simulink model "vipstabilize_fixpt_rowmajor"  (R2015b)
settings: Solver=FixedStepDiscrete  StartTime=0.0  StopTime=inf  RelTol=1e-3
undefined symbols (not defined in the file or in its folder): gray
libraries: visiontextngfix x3, visiongeotforms x2, visionsinks x2, vipmisc x1, dspvision x1, visionanalysis x1
Description:
  | Image stabilization demo.
settings Model: Tag="0  0  0  0  0  1"  FPTRunName=Active  ExtModeAutoUpdateStatusClock=off  Creator=The MathWorks, Inc.  LastModifiedBy=The MathWorks, Inc.
settings DataIOCC: SaveFormat=Array  SaveOutput=off  SaveTime=off  SignalLoggingName=logsOut
settings OptimizationCC: ExpressionDepthLimit=2147483647  InitFltsAndDblsToZero=on  BufferReusableBoundary=off
settings DebuggingCC: UnderspecifiedInitializationDetection=Classic  MergeDetectMultiDrivingBlocksExec=none  CheckExecutionContextPreStartOutputMsg=on  CheckExecutionContextRuntimeOutputMsg=on  SignalResolutionControl=TryResolveAllWithWarning  InheritedTsInSrcMsg=none  MultiTaskDSMMsg=warning  SigSpecEnsureSampleTimeMsg=none  ParameterPrecisionLossMsg=none  UnderSpecifiedDataTypeMsg=error  FcnCallInpInsideContextMsg=UseLocalSettings  BusObjectLabelMismatch=none  StateNameClashWarn=warning  StrictBusMsg=None
settings HardwareCC: ProdBitPerLong=40  ProdBitPerPointer=32  ProdLargestAtomicInteger=Integer  ProdLargestAtomicFloat=None  ProdWordSize=32  ProdHWDeviceType=TI C6000  TargetBitPerLong=64  TargetBitPerPointer=64  TargetLongLongMode=on  TargetIntDivRoundTo=Zero  TargetEndianess=LittleEndian  TargetWordSize=64  TargetHWDeviceType=MATLAB Host  ProdEqTarget=off
settings ModelReferenceCC: UpdateModelReferenceTargets=IfOutOfDate
settings GRTTargetCC: TargetFcnLib=ansi_tfl_tmw_new.mat  GeneratePreprocessorConditionals=Disable all  CombineOutputUpdateFcns=off  GRTInterface=on
settings ConfigComp: CovModelRefEnable=Off

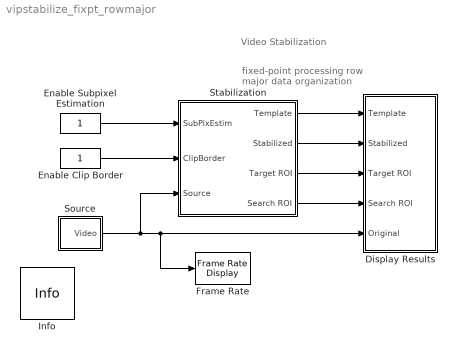
== system vipstabilize_fixpt_rowmajor ==
  note: Video Stabilization
  note: fixed-point processing
      | row major data organization
  Display Results : Subsystem
  Enable Clip Border : Constant  VectorParams1D=off  OutDataTypeStr=boolean
  Enable Subpixel Estimation : Constant  VectorParams1D=off  OutDataTypeStr=boolean
  Frame Rate : visionsinks/Frame Rate Display  UpdateRate=10
  Info : vipmisc/Info  SystemSampleTime=-1
  Source : Subsystem
  Stabilization : Subsystem  mask(Stabilization){template_orig=fliplr([109 100]), template_size=fliplr([18 22]), search_border=fliplr([10 15])}
      mask prompts: template_orig "Upper left corner of the template [x y]:"; template_size "Template size [height width]:"; search_border "Search border [num_rows num_cols]:"
      mask help:
      | Remove motion from the input video signal.
      |
      | Use Upper left corner of template and Template size parameters to define the location and size of the target on the first frame of the input video.  Use Search border to define size of the search region around the target.
      |
      | Note:  You can right-click on Stabilization subsystem and select "Look Under Mask" to explore the design of the underlying algorithm.
      mask init:
      | pos.template_orig = fliplr(template_orig);
      | pos.template_size = template_size;
      | pos.search_border = search_border;
      | pos.template_center = floor((template_size-1)/2);
      | pos.template_center_pos = pos.template_orig + ...
      |     pos.template_center - 1;
      mask Help: Demo subsystem in support of the Video Stabilization demo.  You can right-click on Stabilization subsystem and select "Look Under Mask" to explore the design of the underlying algorithm.
  wires:
  Source/1(Video) -> Frame Rate/1, Display Results/5(Original), Stabilization/3(Source)
  Stabilization/1(Template) -> Display Results/1(Template)
  Stabilization/2(Stabilized) -> Display Results/2(Stabilized)
  Enable Subpixel Estimation/1 -> Stabilization/1(SubPixEstim)
  Enable Clip Border/1 -> Stabilization/2(ClipBorder)
  Stabilization/3(Target ROI) -> Display Results/3(Target ROI)
  Stabilization/4(Search ROI) -> Display Results/4(Search ROI)

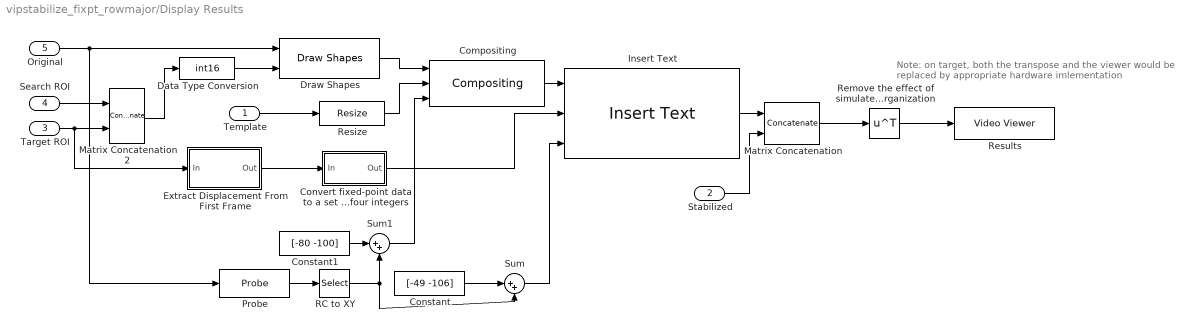
== system vipstabilize_fixpt_rowmajor/Display Results ==
  note: Note: on target, both the transpose and the viewer
      | would be replaced by appropriate hardware imlementation
  Template : Inport
  Stabilized : Inport  Port=2
  Target ROI : Inport  Port=3
  Search ROI : Inport  Port=4
  Original : Inport  Port=5
  Compositing : visiontextngfix/Compositing  operation=Binary mask  bFacSrc=Specify via dialog  mFacSrc=Specify via dialog  bFactor=1  mFactor=1  source=Input port  coordinates=[160 220]  prodOutputMode=Binary point scaling  prodOutputWordLength=32  prodOutputFracLength=10  roundingMode=Floor  overflowMode=off
  Constant : Constant  Value=[-49 -106]  OutDataTypeStr=int16
  Constant1 : Constant  Value=[-80 -100]  OutDataTypeStr=int16
  Convert fixed-point data to a set of four integers : Subsystem
  Data Type Conversion : DataTypeConversion  OutDataTypeStr=int16
  Draw Shapes : visiontextngfix/Draw Shapes  shape=Rectangles  fill=off  lineWidth=1  fillClrSource=Specify via dialog  display=White  intensity=200  color=[200 255 100]  opacity=0.6  viewport=Entire image  antialiasing=off  inType=Intensity  imagePorts=One multidimensional signal  prodOutputMode=Binary point scaling  prodOutputWordLength=32  prodOutputFracLength=14  memoryMode=Specify word length  memoryWordLength=16  memoryFracLength=15  roundingMode=Floor  overflowMode=off
  Extract Displacement From First Frame : Subsystem
  Insert Text : visiontextngfix/Insert Text  inputType=Obsolete  theText='(%+03d.%02d,%+03d.%02d)'  getTextLocFrom=Input port  textLoc=[214 191]  getTextColorFrom=Specify via dialog  textColor=255  getTextIntensityFrom=Specify via dialog  textIntensity=255  getTextOpacityFrom=Specify via dialog  textOpacity=1.0  dummyVar2=0  dummyVar3=0  dummyVar4=0  imagePorts=One multidimensional signal  isInputTransposed=on  fontFace=LucidaTypewriterRegular  dummyVar1=0  blockFontSize=14  antiAliased=on
  Matrix Concatenation : Concatenate  Mode=Multidimensional array
  Matrix Concatenation2 : Concatenate  Mode=Multidimensional array
  Probe : Probe  ProbeWidth=off  ProbeSampleTime=off  ProbeComplexSignal=off  ProbeSignalDimensions=on  ProbeDimensionsDataType=int16
  RC to XY : Selector  IndexOptions=Index vector (dialog)  Indices=[2 1]  OutputSizes=1
  Remove the effect of simulated row major data organization : Math  Operator=transpose  SaturateOnIntegerOverflow=on
  Resize : visiongeotforms/Resize  specify=Output size as a percentage of input size  rfactor=300  outCols=25  outRows=25  outRowsCols=[25 35]  interp_method=Nearest neighbor  antialias=off  useROI=off  roiFlag=off  prodOutputMode=Binary point scaling  prodOutputWordLength=32  prodOutputFracLength=10  roundingMode=Nearest  overflowMode=on
  Results : visionsinks/Video Viewer  inputType=Obsolete7b  imagePorts=One multidimensional signal  useColorMap=off  colormapValue=gray(256)  specRange=off  minInputVal=0  maxInputVal=255  FigPos=[97 364 640 263]  AxisZoom=on  trueSizedOnce=on  OpenAtMdlStart=on  DefaultConfigurationName=vipscopes.VideoViewerScopeCfg
  Sum : Sum  Inputs=|++
  Sum1 : Sum  Inputs=|++
  wires:
  Remove the effect of simulated row major data organization/1 -> Results/1
  RC to XY/1 -> Sum/2, Sum1/2
  Constant/1 -> Sum/1
  Sum/1 -> Insert Text/3
  Probe/1 -> RC to XY/1
  Sum1/1 -> Compositing/3
  Constant1/1 -> Sum1/1
  Template/1 -> Resize/1
  Compositing/1 -> Insert Text/1
  Insert Text/1 -> Matrix Concatenation/1
  Resize/1 -> Compositing/2
  Stabilized/1 -> Matrix Concatenation/2
  Draw Shapes/1 -> Compositing/1
  Matrix Concatenation/1 -> Remove the effect of simulated row major data organization/1
  Convert fixed-point data to a set of four integers/1(Out) -> Insert Text/2
  Matrix Concatenation2/1 -> Data Type Conversion/1
  Original/1 -> Probe/1, Draw Shapes/1
  Extract Displacement From First Frame/1(Out) -> Convert fixed-point data to a set of four integers/1(In)
  Search ROI/1 -> Matrix Concatenation2/1
  Target ROI/1 -> Matrix Concatenation2/2, Extract Displacement From First Frame/1(In)
  Data Type Conversion/1 -> Draw Shapes/2

== system vipstabilize_fixpt_rowmajor/Source ==
  From Multimedia File : dspvision/From Multimedia File  inputFilename=shaky_car.avi  loop=on  numPlays=inf  outputStreams=Video and audio  videoDataType=uint8  audioDataType=int16  inheritSampleTime=on  userDefinedSampleTime=1/30  noAudioOutput=off  isIntensityVideo=off  fourcc=Intensity  colorVideoFormat=Separate color signals  outputEOF=off  dataOrg=Column-major  audioFrameSize=1024  computeAudioFrameSize=off  outSamplingMode=Frame based
  Simulate row major data to ease implementation on hardware : Math  Operator=transpose  SaturateOnIntegerOverflow=on
  Video : Outport
  wires:
  Simulate row major data to ease implementation on hardware/1 -> Video/1
  From Multimedia File/1 -> Simulate row major data to ease implementation on hardware/1

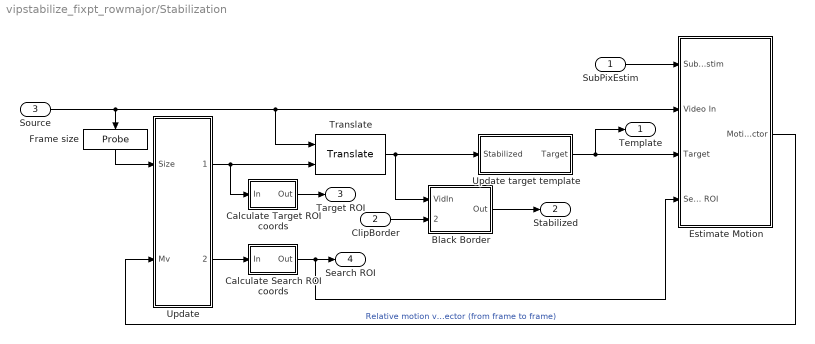
== system vipstabilize_fixpt_rowmajor/Stabilization ==
  SubPixEstim : Inport
  ClipBorder : Inport  Port=2
  Source : Inport  Port=3
  Black Border : Subsystem
  Calculate Search ROI coords : Subsystem
  Calculate Target ROI coords : Subsystem
  Estimate Motion : Subsystem
  Frame size : Probe  ProbeWidth=off  ProbeSampleTime=off  ProbeComplexSignal=off  ProbeSignalDimensions=on  ProbeDimensionsDataType=int16
  Translate : visiongeotforms/Translate  outSizeT=Same as input image  src_trans=Input port  translation="[1.5  2.3]"  maxOffset=[8 10]  fillVal=0  interpMethod=Bilinear  firstCoeffMode=Binary point scaling  firstCoeffWordLength=16  firstCoeffFracLength=6  prodOutputMode=Binary point scaling  prodOutputWordLength=32  prodOutputFracLength=20  roundingMode=Floor  overflowMode=off
  Update : Subsystem
  Update target template : Subsystem
  Template : Outport
  Stabilized : Outport  Port=2
  Target ROI : Outport  Port=3
  Search ROI : Outport  Port=4
  wires:
  Calculate Target ROI coords/1(Out) -> Target ROI/1
  Calculate Search ROI coords/1(Out) -> Search ROI/1, Estimate Motion/4(Search ROI)
  ClipBorder/1 -> Black Border/2(ClipBorder)
  Black Border/1(Out) -> Stabilized/1
  SubPixEstim/1 -> Estimate Motion/1(SubPixEstim)
  Frame size/1 -> Update/1(Size)
  Estimate Motion/1(Motion vector) -> Update/2(Mv)  "Relative motion vector (from frame to frame)"
  Translate/1 -> Update target template/1(Stabilized), Black Border/1(VidIn)
  Source/1 -> Translate/1, Estimate Motion/2(Video In), Frame size/1
  Update target template/1(Target) -> Template/1, Estimate Motion/3(Target)
  Update/2(Location) -> Calculate Search ROI coords/1(In)
  Update/1(Offset) -> Translate/2, Calculate Target ROI coords/1(In)

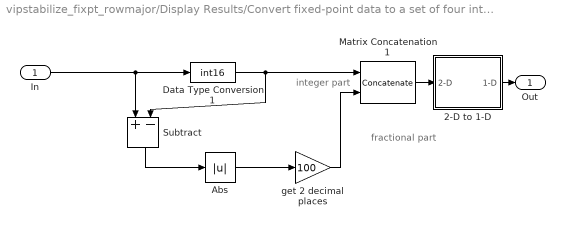
== system vipstabilize_fixpt_rowmajor/Display Results/Convert fixed-point data to a set of four integers ==
  note: integer part
  note: fractional
      | part
  In : Inport
  2-D to 1-D : Subsystem
  Abs : Abs
  Data Type Conversion1 : DataTypeConversion  OutDataTypeStr=int16  RndMeth=Zero
  Matrix Concatenation1 : Concatenate  Mode=Multidimensional array
  Subtract : Sum  Inputs=+-  OutDataTypeStr=Inherit: Same as first input
  get 2 decimal places : Gain  Gain=100  OutDataTypeStr=fixdt(1,16,0)  SaturateOnIntegerOverflow=on
  Out : Outport
  wires:
  Matrix Concatenation1/1 -> 2-D to 1-D/1(2-D)
  Data Type Conversion1/1 -> Matrix Concatenation1/1, Subtract/2
  Subtract/1 -> Abs/1
  Abs/1 -> get 2 decimal places/1
  In/1 -> Data Type Conversion1/1, Subtract/1
  2-D to 1-D/1(1-D) -> Out/1
  get 2 decimal places/1 -> Matrix Concatenation1/2

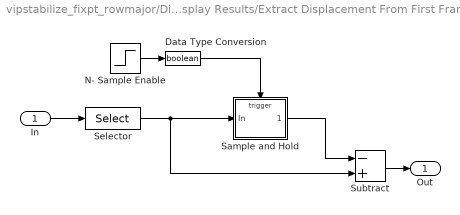
== system vipstabilize_fixpt_rowmajor/Display Results/Extract Displacement From First Frame ==
  In : Inport
  Data Type Conversion : DataTypeConversion  OutDataTypeStr=boolean
  N- Sample Enable : Step  Time=0
  Sample and Hold : Subsystem  TreatAsAtomicUnit=on  mask{initCond=0}
      mask prompts: initCond "Initial Condition"
  Selector : Selector  NumberOfDimensions=2  InputPortWidth=3  IndexOptions=Index vector (dialog),Index vector (dialog)  Indices=1,[1 2]  OutputSizes=1,1
  Subtract : Sum  Inputs=-+
  Out : Outport
  wires:
  Data Type Conversion/1 -> Sample and Hold/Trigger
  In/1 -> Selector/1
  Selector/1 -> Subtract/2, Sample and Hold/1(In)
  Subtract/1 -> Out/1
  Sample and Hold/1(" ") -> Subtract/1
  N- Sample Enable/1 -> Data Type Conversion/1

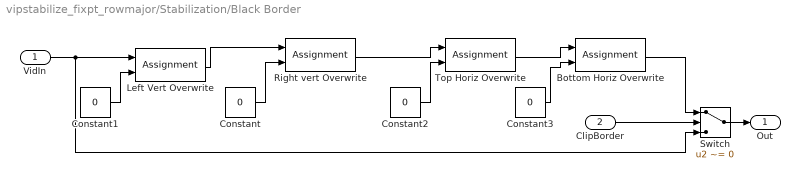
== system vipstabilize_fixpt_rowmajor/Stabilization/Black Border ==
  VidIn : Inport
  ClipBorder : Inport  Port=2
  Bottom Horiz Overwrite : Assignment  NumberOfDimensions=2  IndexOptions=Index vector (dialog),Assign all  Indices=[320-(pos.search_border(2)+4):320],[320-(pos.search_border(2)+4):320]  OutputSizes=1,1
  Constant{,1..3} (4 alike) : Constant  Value=0  OutDataTypeStr=uint8
  Left Vert Overwrite : Assignment  NumberOfDimensions=2  IndexOptions=Assign all,Index vector (dialog)  Indices=1:end,1:(pos.search_border(2)+4)  OutputSizes=1,1
  Right vert Overwrite : Assignment  NumberOfDimensions=2  IndexOptions=Assign all,Index vector (dialog)  Indices=1:end,[240-(pos.search_border(2)+4):240]  OutputSizes=1,1
  Switch : Switch  Criteria=u2 ~= 0  ZeroCross=off
  Top Horiz Overwrite : Assignment  NumberOfDimensions=2  IndexOptions=Index vector (dialog),Assign all  Indices=[1:pos.search_border(1)+4],[320-(pos.search_border(2)+4):320]  OutputSizes=1,1
  Out : Outport
  wires:
  VidIn/1 -> Switch/3, Left Vert Overwrite/1
  Left Vert Overwrite/1 -> Right vert Overwrite/1
  Right vert Overwrite/1 -> Top Horiz Overwrite/1
  Top Horiz Overwrite/1 -> Bottom Horiz Overwrite/1
  ClipBorder/1 -> Switch/2
  Bottom Horiz Overwrite/1 -> Switch/1
  Switch/1 -> Out/1
  Constant1/1 -> Left Vert Overwrite/2
  Constant/1 -> Right vert Overwrite/2
  Constant2/1 -> Top Horiz Overwrite/2
  Constant3/1 -> Bottom Horiz Overwrite/2

== system vipstabilize_fixpt_rowmajor/Stabilization/Calculate Search ROI coords ==
  In : Inport
  Constant : Constant  Value=fliplr(pos.template_size + 2*pos.search_border)  VectorParams1D=off  OutDataTypeStr=fixdt(1,16,6)
  Flip : Selector  NumberOfDimensions=2  IndexOptions=Index vector (dialog),Index vector (dialog)  Indices=1,[2 1]  OutputSizes=1,1
  Matrix Concatenation : Concatenate  Mode=Multidimensional array  ConcatenateDimension=2
  Out : Outport
  wires:
  Flip/1 -> Matrix Concatenation/1
  In/1 -> Flip/1
  Constant/1 -> Matrix Concatenation/2
  Matrix Concatenation/1 -> Out/1

== system vipstabilize_fixpt_rowmajor/Stabilization/Calculate Target ROI coords ==
  In : Inport
  Constant1 : Constant  Value=fliplr(pos.template_size )  VectorParams1D=off  OutDataTypeStr=Inherit: Inherit via back propagation
  Flip : Selector  NumberOfDimensions=2  IndexOptions=Index vector (dialog),Index vector (dialog)  Indices=1,[2 1]  OutputSizes=1,1
  Matrix Concatenation1 : Concatenate  Mode=Multidimensional array  ConcatenateDimension=2
  Sum2 : Sum  Inputs=|-+
  idx3 : Constant  Value=pos.template_orig  VectorParams1D=off  OutDataTypeStr=fixdt(1,16,6)
  Out : Outport
  wires:
  Flip/1 -> Matrix Concatenation1/1
  Matrix Concatenation1/1 -> Out/1
  In/1 -> Sum2/1
  Constant1/1 -> Matrix Concatenation1/2
  Sum2/1 -> Flip/1
  idx3/1 -> Sum2/2

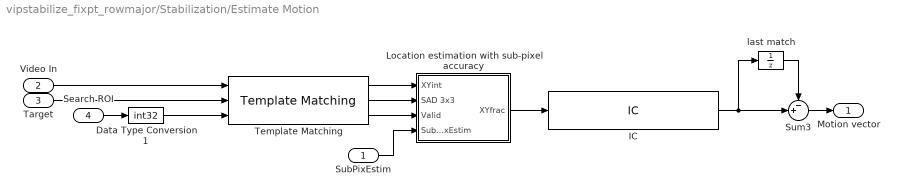
== system vipstabilize_fixpt_rowmajor/Stabilization/Estimate Motion ==
  SubPixEstim : Inport
  Video In : Inport  Port=2
  Target : Inport  Port=3
  Search ROI : Inport  Port=4
  Data Type Conversion1 : DataTypeConversion  OutDataTypeStr=int32  RndMeth=Zero
  IC : InitialCondition  Value=fliplr(pos.template_center_pos)
  Location estimation with sub-pixel accuracy : Subsystem
  Sum3 : Sum  Inputs=-+|  OutDataTypeStr=fixdt(1,16,6)
  Template Matching : visionanalysis/Template Matching  metric=Sum of absolute differences  output=Best match location  method=Exhaustive  nMetric=on  nSize=3  roi=on  roiValid=off  outputMode=Binary point scaling  outputWordLength=16  outputFracLength=-2  accumMode=Binary point scaling  accumWordLength=16  accumFracLength=-2  prodOutputMode=Binary point scaling  prodOutputWordLength=32  prodOutputFracLength=0  roundingMode=Floor  overflowMode=off
  last match : UnitDelay  InitialCondition=fliplr(pos.template_center_pos)  SampleTime=-1
  Motion vector : Outport
  wires:
  Sum3/1 -> Motion vector/1
  Target/1 -> Template Matching/2
  Template Matching/1 -> Location estimation with sub-pixel accuracy/1(XYint)
  Template Matching/2 -> Location estimation with sub-pixel accuracy/2(SAD 3x3)
  Template Matching/3 -> Location estimation with sub-pixel accuracy/3(Valid)
  Video In/1 -> Template Matching/1
  SubPixEstim/1 -> Location estimation with sub-pixel accuracy/4(SubPixEstim)
  Search ROI/1 -> Data Type Conversion1/1
  Data Type Conversion1/1 -> Template Matching/3
  Location estimation with sub-pixel accuracy/1(XYfrac) -> IC/1
  IC/1 -> Sum3/2, last match/1
  last match/1 -> Sum3/1

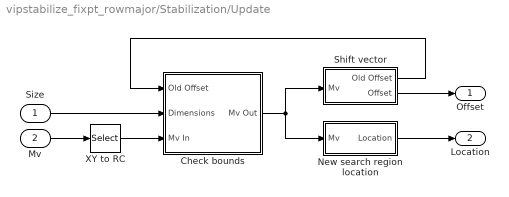
== system vipstabilize_fixpt_rowmajor/Stabilization/Update ==
  Size : Inport
  Mv : Inport  Port=2
  Check bounds : Subsystem
  New search region location : Subsystem
  Shift vector : Subsystem
  XY to RC : Selector  NumberOfDimensions=2  IndexOptions=Index vector (dialog),Index vector (dialog)  Indices=1,[2 1]  OutputSizes=1,1
  Offset : Outport
  Location : Outport  Port=2
  wires:
  Shift vector/1(Old Offset) -> Check bounds/1(Old Offset)
  Mv/1 -> XY to RC/1
  New search region location/1(Location) -> Location/1
  Shift vector/2(Offset) -> Offset/1
  Size/1 -> Check bounds/2(Dimensions)
  Check bounds/1(Mv Out) -> Shift vector/1(Mv), New search region location/1(Mv)
  XY to RC/1 -> Check bounds/3(Mv In)

== system vipstabilize_fixpt_rowmajor/Stabilization/Update target template ==
  note: cut out new template
  Stabilized : Inport
  Delay : UnitDelay  SampleTime=-1
  Selector : Selector  NumberOfDimensions=2  InputPortWidth=3  IndexOptions=Index vector (dialog),Index vector (dialog)  Indices=pos.template_orig(1)-1 : pos.template_orig(1)+pos.template_size(1)-2,pos.template_orig(2)-1 : pos.template_orig(2)+pos.template_size(2)-2  OutputSizes=1,1
  Target : Outport
  wires:
  Delay/1 -> Target/1
  Stabilized/1 -> Selector/1
  Selector/1 -> Delay/1

== system vipstabilize_fixpt_rowmajor/Display Results/Convert fixed-point data to a set of four integers/2-D to 1-D ==
  2-D : Inport
  Frame Conversion : FrameConversion  InheritSamplingMode=off  OutFrame=Sample-based
  Reshape : Reshape
  1-D : Outport
  wires:
  2-D/1 -> Frame Conversion/1
  Frame Conversion/1 -> Reshape/1
  Reshape/1 -> 1-D/1

== system vipstabilize_fixpt_rowmajor/Display Results/Extract Displacement From First Frame/Sample and Hold ==
  In : Inport
  Trigger : TriggerPort  ZeroCross=off
  " " : Outport  InitialOutput=initCond
  wires:
  In/1 -> " "/1

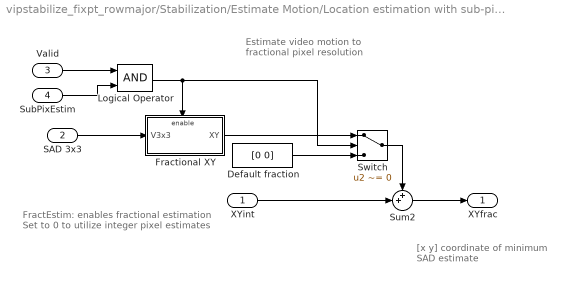
== system vipstabilize_fixpt_rowmajor/Stabilization/Estimate Motion/Location estimation with sub-pixel accuracy ==
  note: [x y] coordinate of
      | minimum SAD estimate
  note: FractEstim: enables fractional estimation
      | Set to 0 to utilize integer pixel estimates
  note: Estimate video motion to
      | fractional pixel resolution
  XYint : Inport
  SAD 3x3 : Inport  Port=2
  Valid : Inport  Port=3
  SubPixEstim : Inport  Port=4
  Default fraction : Constant  Value=[0 0]  VectorParams1D=off  OutDataTypeStr=fixdt(1,8,6)
  Fractional XY : Subsystem  TreatAsAtomicUnit=on
  Logical Operator : Logic  AllPortsSameDT=off  OutDataTypeStr=boolean
  Sum2 : Sum  Inputs=++|  OutDataTypeStr=fixdt(1,16,6)
  Switch : Switch  Criteria=u2 ~= 0
  XYfrac : Outport
  wires:
  XYint/1 -> Sum2/2
  Fractional XY/1(XY) -> Switch/1
  Switch/1 -> Sum2/1
  Default fraction/1 -> Switch/3
  Sum2/1 -> XYfrac/1
  SAD 3x3/1 -> Fractional XY/1(V3x3)
  Logical Operator/1 -> Switch/2, Fractional XY/Enable
  Valid/1 -> Logical Operator/1
  SubPixEstim/1 -> Logical Operator/2

== system vipstabilize_fixpt_rowmajor/Stabilization/Update/Check bounds ==
  Old Offset : Inport
  Dimensions : Inport  Port=2
  Mv In : Inport  Port=3
  Bounds Test : Subsystem
  Constant : Constant  Value=0  OutDataTypeStr=fixdt(1,16,6)
  Switch : Switch  Criteria=u2 ~= 0  ZeroCross=off
  Mv Out : Outport
  wires:
  Mv In/1 -> Bounds Test/1(new_rel), Switch/1  "D_i"
  Switch/1 -> Mv Out/1
  Dimensions/1 -> Bounds Test/3(dim)
  Constant/1 -> Switch/3
  Bounds Test/1(inbounds) -> Switch/2
  Old Offset/1 -> Bounds Test/2(old_abs)

== system vipstabilize_fixpt_rowmajor/Stabilization/Update/New search region location ==
  note: This loop accumulates relative motion vector shifts
  note: Predict new search region location
  Mv : Inport
  Sum2 : Sum  Inputs=++|  RndMeth=Nearest  LockScale=on
  Svi : UnitDelay  InitialCondition=pos.template_orig - pos.search_border - 1  SampleTime=-1
  Location : Outport
  wires:
  Mv/1 -> Sum2/2
  Sum2/1 -> Svi/1
  Svi/1 -> Location/1, Sum2/1  "Upper left corner of the search region"

== system vipstabilize_fixpt_rowmajor/Stabilization/Update/Shift vector ==
  note: this loop keeps track of the absolute shift of the target
  Mv : Inport
  Sum4 : Sum  Inputs=+-|  OutDataTypeStr=fixdt(1,16,6)
  Tvi : UnitDelay  SampleTime=-1
  Old Offset : Outport
  Offset : Outport  Port=2
  wires:
  Mv/1 -> Sum4/2
  Tvi/1 -> Old Offset/1, Sum4/1
  Sum4/1 -> Offset/1, Tvi/1

== system vipstabilize_fixpt_rowmajor/Stabilization/Estimate Motion/Location estimation with sub-pixel accuracy/Fractional XY ==
  note: Ax=b
  V3x3 : Inport
  Enable : EnablePort  StatesWhenEnabling=reset  PropagateVarSize=During execution  ZeroCross=off
  Multiply : Product  Inputs=**  Multiplication=Matrix(*)  OutDataTypeStr=fixdt(1,16,-1)
  Reshape : Reshape  OutputDimensionality=Column vector (2-D)
  Set deriv of quadratic to zero in 2-D : Subsystem
  pinv(X) : Constant  Value=[-4 8 -4 8 20 8 -4 8 -4;-6 -6 -6 0 0 0 6 6 6;-6 0 6 -6 0 6 -6 0 6;9 0 -9 0 0 0 -9 0 9;6 6 6 -12 -12 -12 6 6 6;6 -12 6 6 -12 6 6 -12 6]/36  VectorParams1D=off  OutDataTypeStr=fixdt(1,16)
  XY : Outport
  wires:
  pinv(X)/1 -> Multiply/1
  Multiply/1 -> Set deriv of quadratic to zero in 2-D/1(A)
  V3x3/1 -> Reshape/1
  Reshape/1 -> Multiply/2
  Set deriv of quadratic to zero in 2-D/1(XY) -> XY/1

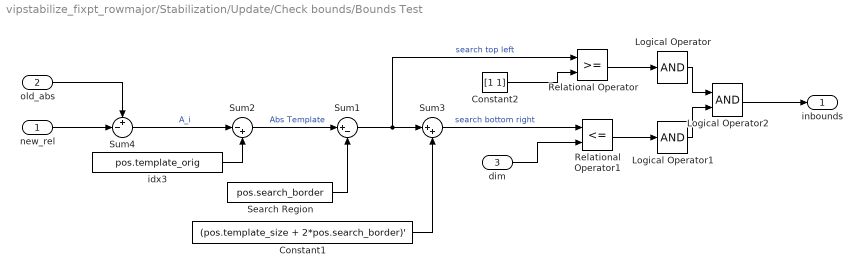
== system vipstabilize_fixpt_rowmajor/Stabilization/Update/Check bounds/Bounds Test ==
  new_rel : Inport
  old_abs : Inport  Port=2
  dim : Inport  Port=3
  Constant1 : Constant  Value=(pos.template_size + 2*pos.search_border)'  OutDataTypeStr=int16
  Constant2 : Constant  Value=[1 1]  OutDataTypeStr=int16
  Logical Operator : Logic  Inputs=1  AllPortsSameDT=off  OutDataTypeStr=boolean
  Logical Operator1 : Logic  Inputs=1  AllPortsSameDT=off  OutDataTypeStr=boolean
  Logical Operator2 : Logic  AllPortsSameDT=off  OutDataTypeStr=boolean
  Relational Operator : RelationalOperator  OutDataTypeStr=boolean
  Relational Operator1 : RelationalOperator  Operator=<=  OutDataTypeStr=boolean
  Search Region : Constant  Value=pos.search_border  OutDataTypeStr=int16
  Sum1 : Sum  Inputs=|+-  OutDataTypeStr=Inherit: Same as first input
  Sum2 : Sum  Inputs=|-+  OutDataTypeStr=int16
  Sum3 : Sum  Inputs=|++  OutDataTypeStr=Inherit: Same as first input
  Sum4 : Sum  Inputs=+-|
  idx3 : Constant  Value=pos.template_orig  OutDataTypeStr=int16
  inbounds : Outport
  wires:
  Logical Operator2/1 -> inbounds/1
  new_rel/1 -> Sum4/2
  old_abs/1 -> Sum4/1
  Sum4/1 -> Sum2/1  "A_i"
  idx3/1 -> Sum2/2
  Sum2/1 -> Sum1/1  "Abs Template"
  Search Region/1 -> Sum1/2
  Sum1/1 -> Sum3/1, Relational Operator/1  "search top left"
  Constant1/1 -> Sum3/2
  Constant2/1 -> Relational Operator/2
  Sum3/1 -> Relational Operator1/1  "search bottom right"
  dim/1 -> Relational Operator1/2
  Relational Operator1/1 -> Logical Operator1/1
  Relational Operator/1 -> Logical Operator/1
  Logical Operator/1 -> Logical Operator2/1
  Logical Operator1/1 -> Logical Operator2/2

== system vipstabilize_fixpt_rowmajor/Stabilization/Estimate Motion/Location estimation with sub-pixel accuracy/Fractional XY/Set deriv of quadratic to zero in 2-D ==
  A : Inport
  Matrix Concatenation : Concatenate  Mode=Multidimensional array  ConcatenateDimension=2
  x offset : Subsystem
  y offset : Subsystem
  XY : Outport
  wires:
  x offset/1(output) -> Matrix Concatenation/1
  y offset/1(output) -> Matrix Concatenation/2
  A/1 -> x offset/1(input), y offset/1(input)
  x offset/2(denominator) -> y offset/2(input1)
  Matrix Concatenation/1 -> XY/1

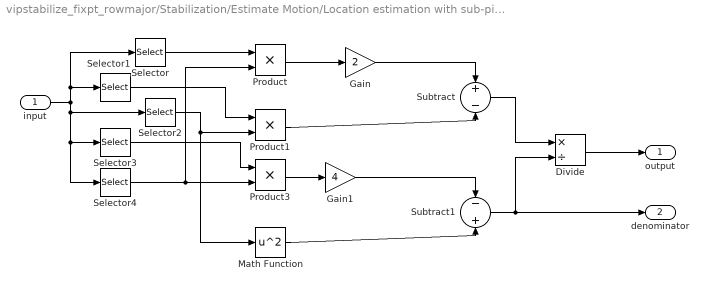
== system vipstabilize_fixpt_rowmajor/Stabilization/Estimate Motion/Location estimation with sub-pixel accuracy/Fractional XY/Set deriv of quadratic to zero in 2-D/x offset ==
  input : Inport
  Divide : Product  Inputs=*/  OutDataTypeStr=fixdt(1,8,6)  SaturateOnIntegerOverflow=on
  Gain : Gain  Gain=2  OutDataTypeStr=Inherit: Same as input
  Gain1 : Gain  Gain=4  OutDataTypeStr=Inherit: Same as input
  Math Function : Math  Operator=square  SaturateOnIntegerOverflow=on  OutDataTypeStr=Inherit: Inherit via internal rule
  Product : Product  RndMeth=Zero
  Product1 : Product  RndMeth=Zero
  Product3 : Product  RndMeth=Zero
  Selector : Selector  IndexMode=Zero-based  IndexOptions=Index vector (dialog)  Indices=(1)  OutputSizes=1
  Selector1 : Selector  IndexMode=Zero-based  IndexOptions=Index vector (dialog)  Indices=(2)  OutputSizes=1
  Selector2 : Selector  IndexMode=Zero-based  IndexOptions=Index vector (dialog)  Indices=(3)  OutputSizes=1
  Selector3 : Selector  IndexMode=Zero-based  IndexOptions=Index vector (dialog)  Indices=(4)  OutputSizes=1
  Selector4 : Selector  IndexMode=Zero-based  IndexOptions=Index vector (dialog)  Indices=(5)  OutputSizes=1
  Subtract : Sum  Inputs=+-  OutDataTypeStr=Inherit: Same as first input
  Subtract1 : Sum  Inputs=-+  OutDataTypeStr=Inherit: Same as first input
  output : Outport
  denominator : Outport  Port=2
  wires:
  Divide/1 -> output/1
  Product/1 -> Gain/1
  Gain/1 -> Subtract/1
  Product1/1 -> Subtract/2
  Product3/1 -> Gain1/1
  Gain1/1 -> Subtract1/1
  Subtract/1 -> Divide/1
  Subtract1/1 -> Divide/2, denominator/1
  input/1 -> Selector/1, Selector1/1, Selector2/1, Selector3/1, Selector4/1
  Math Function/1 -> Subtract1/2
  Selector/1 -> Product/1
  Selector1/1 -> Product1/1
  Selector2/1 -> Product1/2, Math Function/1
  Selector3/1 -> Product3/1
  Selector4/1 -> Product/2, Product3/2

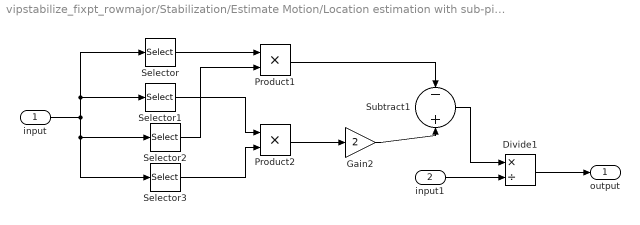
== system vipstabilize_fixpt_rowmajor/Stabilization/Estimate Motion/Location estimation with sub-pixel accuracy/Fractional XY/Set deriv of quadratic to zero in 2-D/y offset ==
  input : Inport
  input1 : Inport  Port=2
  Divide1 : Product  Inputs=*/  OutDataTypeStr=fixdt(1,8,6)  SaturateOnIntegerOverflow=on
  Gain2 : Gain  Gain=2  OutDataTypeStr=Inherit: Same as input
  Product1 : Product  RndMeth=Zero
  Product2 : Product  RndMeth=Zero
  Selector : Selector  IndexMode=Zero-based  IndexOptions=Index vector (dialog)  Indices=(1)  OutputSizes=1
  Selector1 : Selector  IndexMode=Zero-based  IndexOptions=Index vector (dialog)  Indices=(2)  OutputSizes=1
  Selector2 : Selector  IndexMode=Zero-based  IndexOptions=Index vector (dialog)  Indices=(3)  OutputSizes=1
  Selector3 : Selector  IndexMode=Zero-based  IndexOptions=Index vector (dialog)  Indices=(4)  OutputSizes=1
  Subtract1 : Sum  Inputs=-+
  output : Outport
  wires:
  Gain2/1 -> Subtract1/2
  Product2/1 -> Gain2/1
  Divide1/1 -> output/1
  input1/1 -> Divide1/2
  Subtract1/1 -> Divide1/1
  Product1/1 -> Subtract1/1
  input/1 -> Selector/1, Selector1/1, Selector2/1, Selector3/1
  Selector/1 -> Product1/1
  Selector1/1 -> Product2/1
  Selector2/1 -> Product1/2
  Selector3/1 -> Product2/2
